simulink model "model"  (R2023a)
settings: Solver=VariableStepAuto  StartTime=0.0  StopTime=100.0  RelTol=1e-6
values from neighbouring files (symbols this model uses):
  ParSt = MyObject    [main.m]
settings Model: Creator=User  LastModifiedBy=User

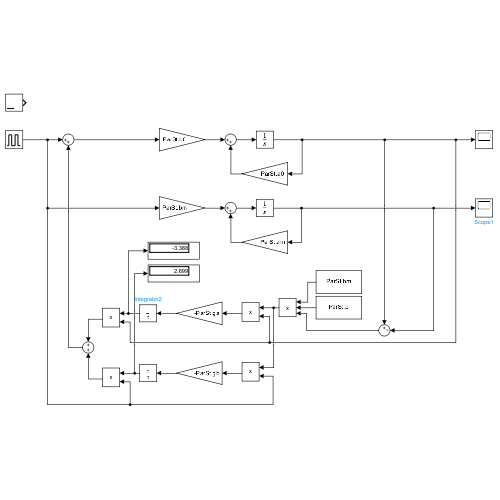
[thumbnail: Simulink's stored preview of the top-level diagram]
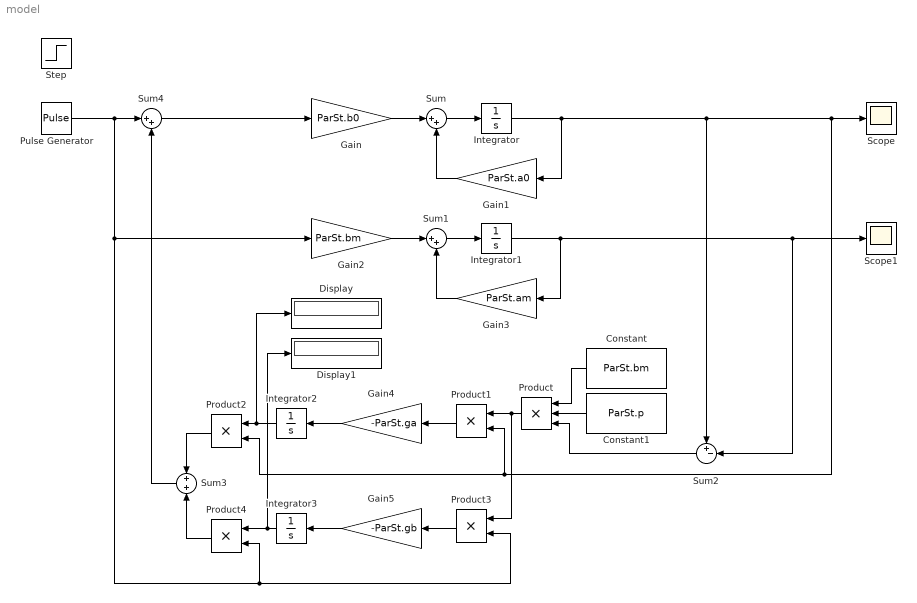
== system model ==
  Constant : Constant  Value=ParSt.bm
  Constant1 : Constant  Value=ParSt.p
  Display : Display
  Display1 : Display
  Gain : Gain  Gain=ParSt.b0
  Gain1 : Gain  Gain=ParSt.a0
  Gain2 : Gain  Gain=ParSt.bm
  Gain3 : Gain  Gain=ParSt.am
  Gain4 : Gain  Gain=-ParSt.ga
  Gain5 : Gain  Gain=-ParSt.gb
  Integrator{,1..3} (4 alike) : Integrator
  Product : Product  Inputs=3
  Product{1..4} (4 alike) : Product
  Pulse Generator : DiscretePulseGenerator  PulseType=Time based  Period=20  PulseWidth=50
  Scope : Scope
  Scope1 : Scope
  Step : Step  Time=0  SampleTime=0
  Sum : Sum  Inputs=|++
  Sum1 : Sum  Inputs=|++
  Sum2 : Sum  Inputs=+-|
  Sum3 : Sum
  Sum4 : Sum  Inputs=|++
  wires:
  Sum/1 -> Integrator/1
  Integrator/1 -> Product1/2, Product2/2, Scope/1, Sum2/1, Gain1/1
  Gain1/1 -> Sum/2
  Gain/1 -> Sum/1
  Gain2/1 -> Sum1/1
  Gain3/1 -> Sum1/2
  Integrator1/1 -> Sum2/2, Scope1/1, Gain3/1
  Sum1/1 -> Integrator1/1
  Constant/1 -> Product/1
  Constant1/1 -> Product/2
  Sum2/1 -> Product/3
  Product/1 -> Product3/1, Product1/1
  Product1/1 -> Gain4/1
  Gain4/1 -> Integrator2/1
  Integrator2/1 -> Display/1, Product2/1
  Product3/1 -> Gain5/1
  Gain5/1 -> Integrator3/1
  Integrator3/1 -> Display1/1, Product4/1
  Product2/1 -> Sum3/1
  Sum4/1 -> Gain/1
  Sum3/1 -> Sum4/2
  Product4/1 -> Sum3/2
  Pulse Generator/1 -> Product3/2, Product4/2, Gain2/1, Sum4/1
